simulink model "flowChart_01"  (R2024a)
settings: Solver=FixedStepDiscrete  StartTime=0.0  StopTime=10.0  FixedStep=.1  RelTol=1e-3
settings Model: Creator=User  LastModifiedBy=User

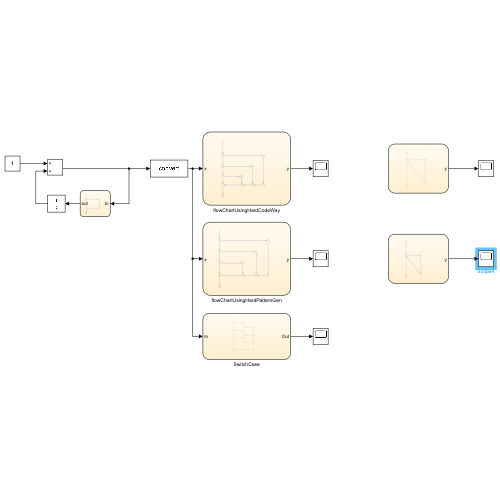
[thumbnail: Simulink's stored preview of the top-level diagram]
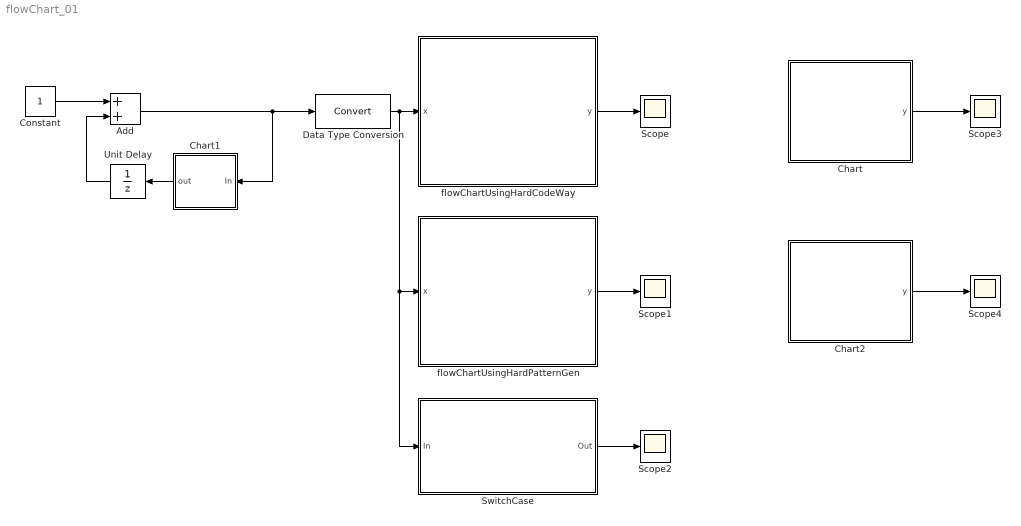
== system flowChart_01 ==
  Add : Sum
  Chart : Stateflow chart  TreatAsAtomicUnit=on
  Chart1 : Stateflow chart  TreatAsAtomicUnit=on
  Chart2 : Stateflow chart  TreatAsAtomicUnit=on
  Constant : Constant
  Data Type Conversion : DataTypeConversion  SaturateOnIntegerOverflow=off  RndMeth=Floor
  Scope{,1..4} (5 alike) : Scope
  SwitchCase : Stateflow chart  TreatAsAtomicUnit=on
  Unit Delay : UnitDelay  SampleTime=-1  HasFrameUpgradeWarning=on
  flowChartUsingHardCodeWay : Stateflow chart  TreatAsAtomicUnit=on
  flowChartUsingHardPatternGen : Stateflow chart  TreatAsAtomicUnit=on
  wires:
  Add/1 -> Data Type Conversion/1, Chart1/1(In)
  flowChartUsingHardCodeWay/1(y) -> Scope/1
  Constant/1 -> Add/1
  Unit Delay/1 -> Add/2
  Data Type Conversion/1 -> SwitchCase/1(In), flowChartUsingHardPatternGen/1(x), flowChartUsingHardCodeWay/1(x)
  Chart1/1(out) -> Unit Delay/1
  flowChartUsingHardPatternGen/1(y) -> Scope1/1
  SwitchCase/1(Out) -> Scope2/1
  Chart/1(y) -> Scope3/1
  Chart2/1(y) -> Scope4/1

== stateflow chart flowChart_01/flowChartUsingHardCodeWay ==
  (default) -> (junction 1)
  (junction 1) -> (junction 5) [order 1] : [x==1]
  (junction 1) -> (junction 7) [order 2]
  (junction 5) -> (junction 12) : {y=1;}
  (junction 7) -> (junction 11) [order 1] : [x==2]
  (junction 7) -> (junction 16) [order 2]
  (junction 11) -> (junction 14) : {y=2;}
  (junction 16) -> (junction 18) [order 1] : [x==3]
  (junction 16) -> (junction 24) [order 2]
  (junction 18) -> (junction 20) : {y=3;}
  (junction 20) -> (junction 24)
  (junction 14) -> (junction 20)
  (junction 12) -> (junction 14)
  (junction 24) -> (junction 27)
  data: x input uint8; y output uint8

== stateflow chart flowChart_01/SwitchCase ==
  note: Do not put any code along
      | the transitions that run
      | down the right side!
  (default) -> (junction 20) : % MBD on the Way
  (junction 20) -> (junction 21) [order 1] : [In == 1]
  (junction 20) -> (junction 24) [order 2]
  (junction 21) -> (junction 22) : {Out=1;}
  (junction 22) -> (junction 23)
  (junction 23) -> (junction 27)
  (junction 24) -> (junction 25) [order 1] : [In == 2]
  (junction 24) -> (junction 28) [order 2]
  (junction 25) -> (junction 26) : {Out=2;}
  (junction 26) -> (junction 27)
  (junction 27) -> (junction 31)
  (junction 28) -> (junction 29) [order 1] : [In == 3]
  (junction 28) -> (junction 32) [order 2] : {Out=9;}
  (junction 29) -> (junction 30) : {Out=3;}
  (junction 30) -> (junction 31)
  (junction 31) -> (junction 33)
  (junction 33) -> (junction 32)
  (junction 32) -> (junction 34)
  data: In input; Out output

== stateflow chart flowChart_01/Chart ==
  (default) -> (junction 8) : % For loop Example
  (junction 8) -> (junction 10) : {i =0;}
  (junction 10) -> (junction 9) [order 1] : [i <5]
  (junction 9) -> (junction 11) : {y = y + 1;}
  (junction 12) -> (junction 10)
  (junction 10) -> (junction 13) [order 2]
  (junction 11) -> (junction 12) : {i = i + 1;}
  data: i local uint8 =0; y output uint8

== stateflow chart flowChart_01/Chart2 ==
  (default) -> (junction 23) : /* while loop Example */
  (junction 23) -> (junction 25)
  (junction 25) -> (junction 24) [order 1] : [i <= 5]
  (junction 26) -> (junction 25)
  (junction 24) -> (junction 26) : {y=y+1;i=i+1;}
  (junction 25) -> (junction 27) [order 2]
  data: i local uint8 =0; y output uint8 =0

== stateflow chart flowChart_01/Chart1 ==
  (default) -> (junction 9) : % reset to zero
  (junction 9) -> (junction 10) [order 1] : [In==3]
  (junction 9) -> (junction 11) [order 2] : {out=In;}
  (junction 10) -> (junction 12) : {out=0;}
  (junction 12) -> (junction 11)
  (junction 11) -> (junction 13)
  data: In input; out output

== stateflow chart flowChart_01/flowChartUsingHardPatternGen ==
  (default) -> (junction 68) : /* if else if else if else */
  (junction 68) -> (junction 69) [order 1] : [x ==1]
  (junction 68) -> (junction 70) [order 2]
  (junction 69) -> (junction 77) : {y=1;}
  (junction 70) -> (junction 71) [order 1] : [x ==2]
  (junction 70) -> (junction 72) [order 2]
  (junction 71) -> (junction 76) : {y=2;}
  (junction 72) -> (junction 73) [order 1] : [x ==3]
  (junction 72) -> (junction 74) [order 2]
  (junction 73) -> (junction 75) : {y=3;}
  (junction 75) -> (junction 74)
  (junction 76) -> (junction 75)
  (junction 77) -> (junction 76)
  (junction 74) -> (junction 78)
  data: x input uint8; y output uint8
